simulink subsystem "Guide_Flight_Path_Energy"  (R2025b)
settings: Solver=VariableStepAuto  StartTime=0.0  StopTime=10.0  RelTol=1e-3
undefined symbols (not defined in the file): alpha, EngineThrustCMD, U1
settings Model: Creator=invrt  LastModifiedBy=Ky Bui

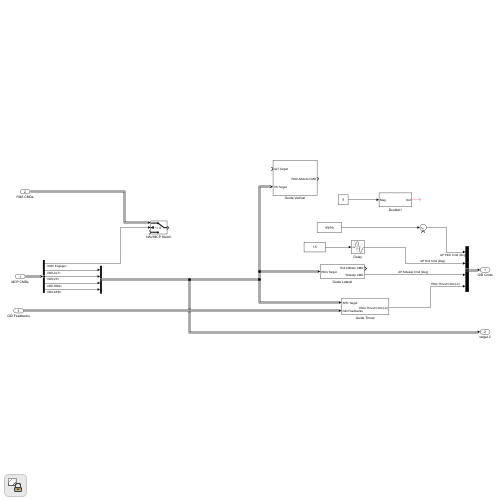
[thumbnail: Simulink's stored preview of the top-level diagram]
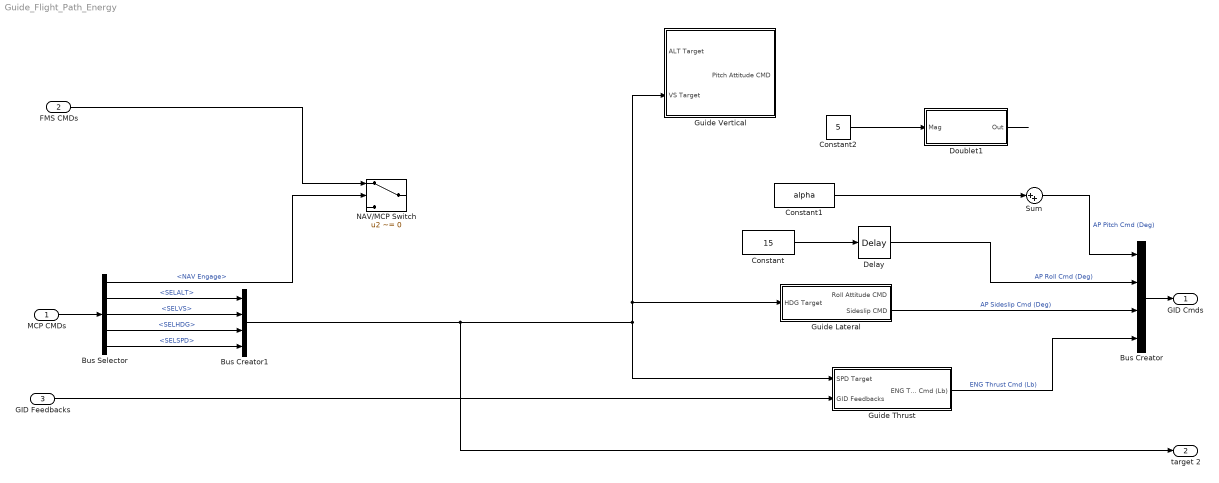
== system Guide_Flight_Path_Energy ==
  MCP CMDs : Inport
  FMS CMDs : Inport  Port=2
  GID Feedbacks : Inport  Port=3
  Bus Creator : BusCreator  Inputs=4
  Bus Creator1 : BusCreator  Inputs=4
  Bus Selector : BusSelector  OutputSignals=NAV Engage,Vert GID Bus.SELALT,Vert GID Bus.SELVS,Lat GID Bus.SELHDG,Spd/Mach GID Bus.SELSPD
  Constant : Constant  Value=15
  Constant1 : Constant  Value=alpha
  Constant2 : Constant  Value=5
  Delay : TransportDelay  DelayTime=5
  Doublet1 : Subsystem
  Guide Lateral : Subsystem
  Guide Thrust : Subsystem
  Guide Vertical : Subsystem
  NAV/MCP Switch : Switch  Criteria=u2 ~= 0  OutDataTypeStr=Inherit: Inherit via back propagation  SaturateOnIntegerOverflow=off
  Sum : Sum  Inputs=|++
  GID Cmds : Outport
  target 2 : Outport  Port=2
  wires:
  Guide Lateral/2(Sideslip CMD) -> Bus Creator/3  "AP Sideslip Cmd (Deg)"
  Bus Creator/1 -> GID Cmds/1
  MCP CMDs/1 -> Bus Selector/1
  Bus Selector/1 -> NAV/MCP Switch/2  "<NAV Engage>"
  Bus Selector/2 -> Bus Creator1/1  "<SELALT>"
  Bus Selector/3 -> Bus Creator1/2  "<SELVS>"
  Bus Selector/4 -> Bus Creator1/3  "<SELHDG>"
  FMS CMDs/1 -> NAV/MCP Switch/1
  Bus Creator1/1 -> Guide Thrust/1(SPD Target), Guide Vertical/2(VS Target), Guide Lateral/1(HDG Target), target 2/1
  GID Feedbacks/1 -> Guide Thrust/2(GID Feedbacks)
  Guide Thrust/1(ENG Thrust Cmd (Lb)) -> Bus Creator/4  "ENG Thrust Cmd (Lb)"
  Bus Selector/5 -> Bus Creator1/4  "<SELSPD>"
  Constant2/1 -> Doublet1/1(Mag)
  Doublet1/1(Out) -> ?
  Sum/1 -> Bus Creator/1  "AP Pitch Cmd (Deg)"
  Constant1/1 -> Sum/1
  Constant/1 -> Delay/1
  Delay/1 -> Bus Creator/2  "AP Roll Cmd (Deg)"

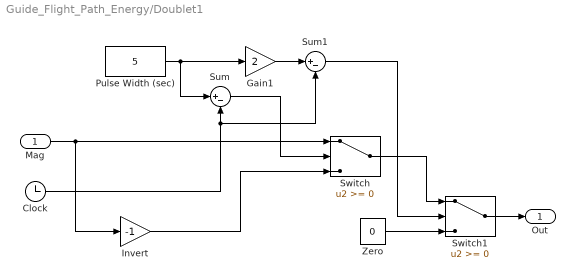
== system Guide_Flight_Path_Energy/Doublet1 ==
  Mag : Inport
  Clock : Clock
  Gain1 : Gain  Gain=2
  Invert : Gain  Gain=-1
  Pulse Width (sec) : Constant  Value=5
  Sum : Sum  Inputs=|+-
  Sum1 : Sum  Inputs=|+-
  Switch : Switch  SaturateOnIntegerOverflow=off  InputSameDT=off
  Switch1 : Switch  SaturateOnIntegerOverflow=off  InputSameDT=off
  Zero : Constant  Value=0
  Out : Outport
  wires:
  Sum1/1 -> Switch1/2
  Gain1/1 -> Sum1/1
  Switch1/1 -> Out/1
  Sum/1 -> Switch/2
  Clock/1 -> Sum/2, Sum1/2
  Zero/1 -> Switch1/3
  Switch/1 -> Switch1/1
  Invert/1 -> Switch/3
  Pulse Width (sec)/1 -> Gain1/1, Sum/1
  Mag/1 -> Invert/1, Switch/1

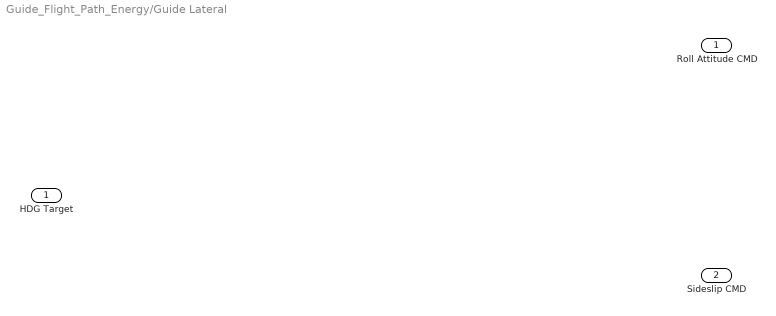
== system Guide_Flight_Path_Energy/Guide Lateral ==
  HDG Target : Inport
  Roll Attitude CMD : Outport
  Sideslip CMD : Outport  Port=2

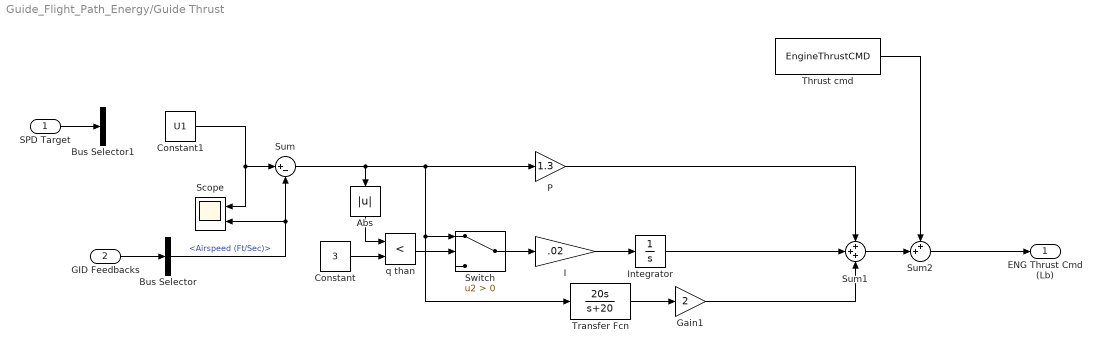
== system Guide_Flight_Path_Energy/Guide Thrust ==
  SPD Target : Inport
  GID Feedbacks : Inport  Port=2
  Abs : Abs  SaturateOnIntegerOverflow=off
  Bus Selector : BusSelector  OutputSignals=Airspeed (Ft/Sec)
  Bus Selector1 : BusSelector  OutputSignals=SELSPD
  Constant : Constant  Value=3
  Constant1 : Constant  Value=U1
  Gain1 : Gain  Gain=2
  I : Gain  Gain=.02
  Integrator : Integrator  LimitOutput=on  UpperSaturationLimit=1  LowerSaturationLimit=-1
  P : Gain  Gain=1.3
  Scope : Scope  NumInputPorts=2
      settings: ActiveDisplayYMinimum=868.72685468796908  ActiveDisplayYMaximum=899.17143805629928  DataLoggingVariableName=ScopeData26
  Sum : Sum  Inputs=|+-
  Sum1 : Sum  Inputs=+++
  Sum2 : Sum  Inputs=++|
  Switch : Switch  Criteria=u2 > Threshold  SaturateOnIntegerOverflow=off  InputSameDT=off
  Thrust cmd : Constant  Value=EngineThrustCMD
  Transfer Fcn : TransferFcn  Numerator=[20 0]  Denominator=[1 20]
  q than : RelationalOperator  Operator=<  OutDataTypeStr=boolean  RndMeth=Simplest  InputSameDT=off
  ENG Thrust Cmd (Lb) : Outport
  wires:
  Integrator/1 -> Sum1/2
  Gain1/1 -> Sum1/3
  Transfer Fcn/1 -> Gain1/1
  I/1 -> Integrator/1
  Abs/1 -> q than/1
  Switch/1 -> I/1
  Constant/1 -> q than/2
  q than/1 -> Switch/2
  Sum/1 -> Abs/1, P/1, Switch/1, Transfer Fcn/1
  Sum2/1 -> ENG Thrust Cmd (Lb)/1
  Thrust cmd/1 -> Sum2/1
  P/1 -> Sum1/1
  Bus Selector/1 -> Scope/2, Sum/2  "<Airspeed (Ft/Sec)>"
  GID Feedbacks/1 -> Bus Selector/1
  SPD Target/1 -> Bus Selector1/1
  Sum1/1 -> Sum2/2
  Constant1/1 -> Scope/1, Sum/1

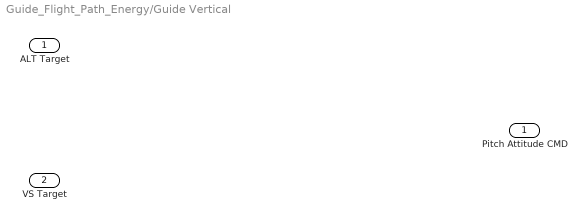
== system Guide_Flight_Path_Energy/Guide Vertical ==
  ALT Target : Inport
  VS Target : Inport  Port=2
  Pitch Attitude CMD : Outport
